simulink model "Test"  (R2014a)
settings: Solver=ode3  StartTime=0.0  StopTime=7  FixedStep=1e-1  RelTol=1e-3
values from neighbouring files (symbols this model uses):
  alphacoeff_xdata = alphacoeff_xdata2    [param.m]
  alphacoeff_yddata = interp1(alphacoeff_xdata,alphacoeff_yddata,alphacoeff_xdata2,'pchip')    [param.m]
libraries: simulink x1
settings Model: Creator=paul  LastModifiedBy=paul

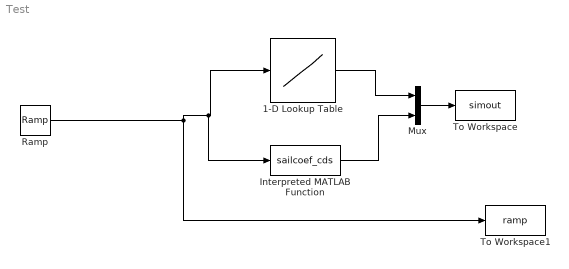
== system Test ==
  1-D Lookup Table : Lookup_n-D  NumberOfTableDimensions=1  BreakpointsForDimension1=alphacoeff_xdata  Table=alphacoeff_yddata  InterpMethod=Cubic spline  RndMeth=Simplest  InputSameDT=on
  Interpreted MATLAB Function : MATLABFcn  MATLABFcn=sailcoef_cds
  Mux : Mux  Inputs=2
  Ramp : simulink/Sources/Ramp  slope=1  start=0  X0=-pi
  To Workspace : ToWorkspace  VariableName=simout  SaveFormat=Timeseries  SampleTime=-1
  To Workspace1 : ToWorkspace  VariableName=ramp  SaveFormat=Timeseries  SampleTime=-1
  wires:
  Ramp/1 -> Interpreted MATLAB Function/1, 1-D Lookup Table/1, To Workspace1/1
  Mux/1 -> To Workspace/1
  1-D Lookup Table/1 -> Mux/1
  Interpreted MATLAB Function/1 -> Mux/2
